simulink model "DCtoACtoDCConverter"  (R2024b)
settings: Solver=VariableStepAuto  StartTime=0.0  StopTime=10.0  RelTol=1e-3
libraries: spsUniversalBridgeLib x2, spsPLL3phLib x1, spsPower3phInstantaneousLib x1, spsPWMGenerator2LevelLib x1, spsThreePhaseSeriesRLCBranchLib x1, spsThreePhaseSeriesRLCLoadLib x1, spsThreePhaseVIMeasurementLib x1, spsThreePhaseBreakerLib x1
settings Model: Creator=Korisnik  LastModifiedBy=Nadir

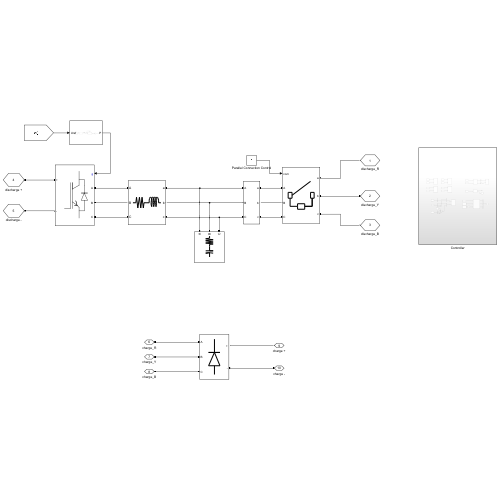
[thumbnail: Simulink's stored preview of the top-level diagram]
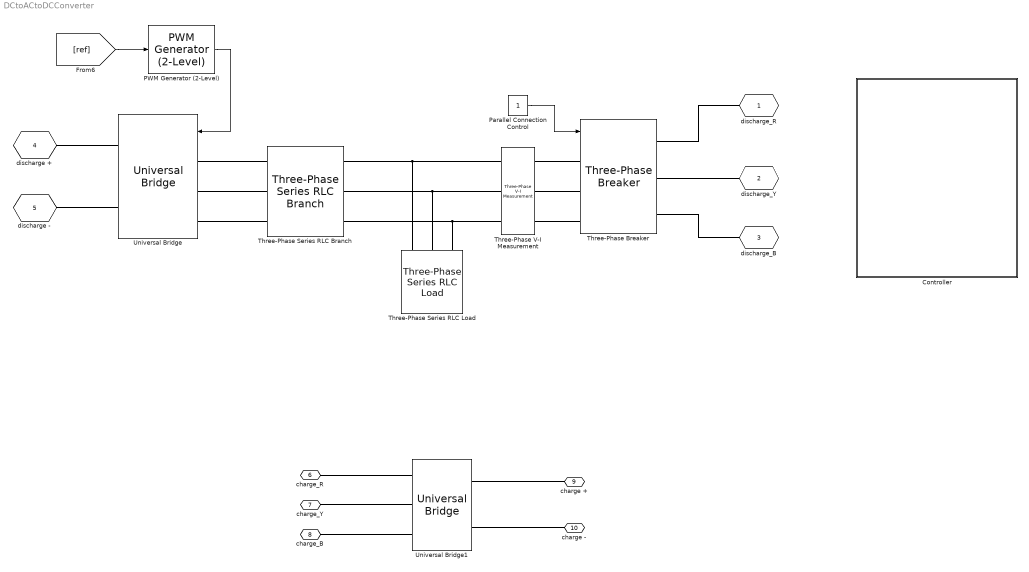
== system DCtoACtoDCConverter ==
  Controller : Subsystem
  PWM Generator (2-Level) : spsPWMGenerator2LevelLib/PWM Generator (2-Level)  ModulatorType=Three-phase bridge (6 pulses)  ModulatorMode=Unsynchronized  Fc=4950  Pc=90  nF=27  MinMax="[ -1  1 ]"  SamplingTechnique=Natural  ModulatingSignals=off  m=0.8  Freq=60  Phase=0  Ts=2.02e-6  ShowCarrierOutport=off
  Parallel Connection Control : Constant
  Three-Phase Series RLC Branch : spsThreePhaseSeriesRLCBranchLib/Three-Phase Series RLC Branch  LConnTagsString=A|B|C  RConnTagsString=A|B|C  BranchType=RL  Resistance=0.004332  Inductance=0.0013789184  Capacitance=1e-6  Measurements=None
  Three-Phase Series RLC Load : spsThreePhaseSeriesRLCLoadLib/Three-Phase Series RLC Load  LConnTagsString=A|B|C  Configuration=Delta  NominalVoltage=380  Vabc=[1e3 1e3 1e3]  Vabcp=[1e3 1e3 1e3]  NominalFrequency=50  UnbalancedPower=off  ActivePower=100  InductivePower=0  CapacitivePower=5000  Pabc=[10e3 9e3 11e3]  QLabc=[100 90 110]  QCabc=[100 90 110]  Pabcp=[10e3 9e3 11e3]  QLabcp=[100 90 110]  QCabcp=[100 90 110]  Measurements=None  LoadType=constant Z
  Three-Phase V-I Measurement : spsThreePhaseVIMeasurementLib/Three-Phase V-I Measurement  VoltageMeasurement=phase-to-phase  SetLabelV=on  LabelV=Vabc_inv  Vpu=off  VpuLL=off  CurrentMeasurement=yes  SetLabelI=on  LabelI=Iabc_inv  Ipu=off  Pbase=100e6  Vbase=500e3  OutputType=Complex  PhasorSimulation=off  PSBequivalent=0
  Three-Phase Breaker : spsThreePhaseBreakerLib/Three-Phase Breaker  InitialState=open  SwitchA=on  SwitchB=on  SwitchC=on  SwitchTimes="[1/60  5/60]"  External=on  BreakerResistance=0.01  SnubberResistance=1e6  SnubberCapacitance=inf  Measurements=None
  Universal Bridge : spsUniversalBridgeLib/Universal Bridge  Arms=3  SnubberResistance=1e6  SnubberCapacitance=inf  Device=IGBT / Diodes  Ron=1e-3  Lon=0  ForwardVoltages="[  0  0  ]"  ForwardVoltage=0  GTOparameters=[ 10e-6 , 20e-6 ]  IGBTparameters=[ 1e-6 , 2e-6 ]  Measurements=None  Measurements_2=None  converterType=Rectifier
  Universal Bridge1 : spsUniversalBridgeLib/Universal Bridge  Arms=3  SnubberResistance=1e5  SnubberCapacitance=inf  Device=Diodes  Ron=1e-3  Lon=0  ForwardVoltages="[  0  0  ]"  ForwardVoltage=0  GTOparameters=[ 10e-6 , 20e-6 ]  IGBTparameters=[ 1e-6 , 2e-6 ]  Measurements=None  Measurements_2=None  converterType=Rectifier
  discharge_R : PMIOPort  Side=Left
  discharge_Y : PMIOPort  Port=2  Side=Left
  discharge_B : PMIOPort  Port=3  Side=Left
  discharge + : PMIOPort  Port=4  Side=Right
  discharge - : PMIOPort  Port=5  Side=Right
  charge_R : PMIOPort  Port=6  Side=Left
  charge_Y : PMIOPort  Port=7  Side=Left
  charge_B : PMIOPort  Port=8  Side=Left
  charge + : PMIOPort  Port=9  Side=Right
  charge - : PMIOPort  Port=10  Side=Right
  wires:
  [ref] -> PWM Generator (2-Level)/1
  PWM Generator (2-Level)/1 -> Universal Bridge/1
  Parallel Connection Control/1 -> Three-Phase Breaker/1
  connections:
  Universal Bridge/RConn1 -- discharge +/RConn1
  discharge -/RConn1 -- Universal Bridge/RConn2
  Universal Bridge/LConn1 -- Three-Phase Series RLC Branch/LConn1
  Three-Phase Series RLC Branch/LConn2 -- Universal Bridge/LConn2
  Three-Phase Series RLC Branch/LConn3 -- Universal Bridge/LConn3
  Three-Phase V-I Measurement/LConn1 -- Three-Phase Series RLC Load/LConn1 -- Three-Phase Series RLC Branch/RConn1
  Three-Phase V-I Measurement/LConn2 -- Three-Phase Series RLC Load/LConn2 -- Three-Phase Series RLC Branch/RConn2
  Three-Phase V-I Measurement/LConn3 -- Three-Phase Series RLC Load/LConn3 -- Three-Phase Series RLC Branch/RConn3
  Three-Phase Breaker/LConn1 -- Three-Phase V-I Measurement/RConn1
  Three-Phase Breaker/LConn2 -- Three-Phase V-I Measurement/RConn2
  Three-Phase Breaker/LConn3 -- Three-Phase V-I Measurement/RConn3
  Three-Phase Breaker/RConn1 -- discharge_R/RConn1
  Three-Phase Breaker/RConn2 -- discharge_Y/RConn1
  Three-Phase Breaker/RConn3 -- discharge_B/RConn1
  charge_R/RConn1 -- Universal Bridge1/LConn1
  charge_Y/RConn1 -- Universal Bridge1/LConn2
  charge_B/RConn1 -- Universal Bridge1/LConn3
  Universal Bridge1/RConn1 -- charge +/RConn1
  Universal Bridge1/RConn2 -- charge -/RConn1

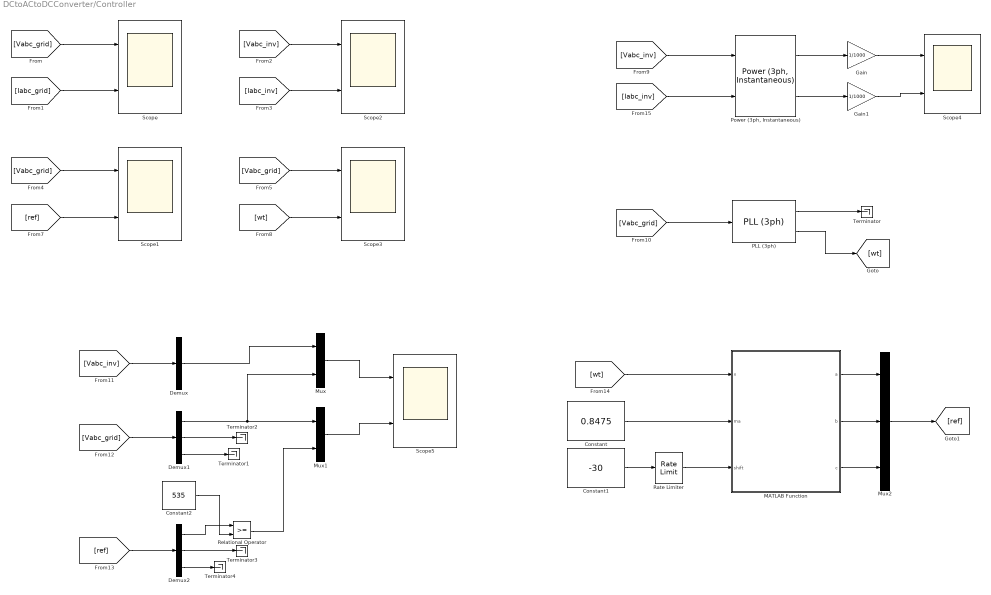
== system DCtoACtoDCConverter/Controller ==
  Constant : Constant  Value=0.8475
  Constant1 : Constant  Value=-30
  Constant2 : Constant  Value=535
  Demux : Demux  Outputs=1
  Demux1 : Demux  Outputs=3
  Demux2 : Demux  Outputs=3
  Gain : Gain  Gain=1/1000
  Gain1 : Gain  Gain=1/1000
  MATLAB Function : MATLAB Function  TreatAsAtomicUnit=on
  Mux : Mux  Inputs=2
  Mux1 : Mux  Inputs=2
  Mux2 : Mux  Inputs=3
  PLL (3ph) : spsPLL3phLib/PLL (3ph)  Fmin=45  Par_Init=[0, 60]  ParK=[180, 3200, 1]  TcD=1e-4  MaxRateChangeFreq=12  FilterCutOffFreq=25  Ts=2.02e-6  AGC=on
  "Power (3ph, Instantaneous)" : spsPower3phInstantaneousLib/Power (3ph, Instantaneous)
  Rate Limiter : RateLimiter  SampleTimeMode=inherited
  Relational Operator : RelationalOperator  OutDataTypeStr=boolean  RndMeth=Simplest  InputSameDT=off
  Scope{,1..5} (6 alike) : Scope  NumInputPorts=2
  Terminator{,1..4} (5 alike) : Terminator
  wires:
  MATLAB Function/3(c) -> Mux2/3
  MATLAB Function/2(b) -> Mux2/2
  Demux1/3 -> Terminator1/1
  Demux2/3 -> Terminator4/1
  Mux/1 -> Scope5/1
  [ref] -> Demux2/1
  Constant2/1 -> Relational Operator/2
  [Iabc_grid] -> Scope/2
  Constant/1 -> MATLAB Function/2(ma)
  Demux1/1 -> Mux/2, Mux1/1
  MATLAB Function/1(a) -> Mux2/1
  [Vabc_grid] -> Demux1/1
  Demux2/1 -> Relational Operator/1
  Constant1/1 -> Rate Limiter/1
  Demux2/2 -> Terminator3/1
  [wt] -> MATLAB Function/1(x)
  Demux/1 -> Mux/1
  Mux1/1 -> Scope5/2
  Demux1/2 -> Terminator2/1
  [Vabc_inv] -> Demux/1
  PLL (3ph)/1 -> Terminator/1
  Rate Limiter/1 -> MATLAB Function/3(shift)
  [Iabc_inv] -> Scope2/2
  [wt] -> Scope3/2
  [Vabc_grid] -> Scope1/1
  [Vabc_grid] -> Scope3/1
  [ref] -> Scope1/2
  Relational Operator/1 -> Mux1/2
  [Vabc_grid] -> PLL (3ph)/1
  [Vabc_inv] -> Scope2/1
  Gain/1 -> Scope4/1
  PLL (3ph)/2 -> [wt]
  "Power (3ph, Instantaneous)"/2 -> Gain1/1
  [Vabc_inv] -> "Power (3ph, Instantaneous)"/1
  "Power (3ph, Instantaneous)"/1 -> Gain/1
  [Iabc_inv] -> "Power (3ph, Instantaneous)"/2
  Mux2/1 -> [ref]
  Gain1/1 -> Scope4/2
  [Vabc_grid] -> Scope/1

== matlab function DCtoACtoDCConverter/Controller/MATLAB Function ==
  data: x input; a output; ma input; shift input; b output; c output
function [a, b, c] = ref_generation(x, ma, shift)

shift_k = shift * pi / 180;
a = (ma * (sin((x) + shift_k)));
b = (ma * (sin((x) + shift_k - (2*pi/3))));
c = (ma * (sin((x) + shift_k + (2*pi/3))));
